simulink model "sim"  (R2020a)
settings: Solver=FixedStepAuto  StartTime=0.0  StopTime=2  FixedStep=0.001  RelTol=1e-3
undefined symbols (not defined in the file): A, B, C, x_0
libraries: simulink_extras x3
settings Model: Creator=Artis  LastModifiedBy=Emil

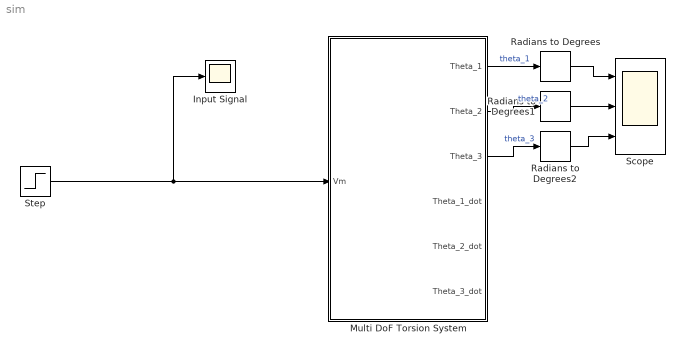
== system sim ==
  Input Signal : Scope
  Multi DoF Torsion System : Subsystem
  Radians to Degrees : simulink_extras/Transformations/Radians to Degrees
  Radians to Degrees1 : simulink_extras/Transformations/Radians to Degrees
  Radians to Degrees2 : simulink_extras/Transformations/Radians to Degrees
  Scope : Scope  NumInputPorts=3
  Step : Step  Before=6  After=0  SampleTime=0
  wires:
  Step/1 -> Multi DoF Torsion System/1(Vm), Input Signal/1
  Radians to Degrees2/1 -> Scope/3
  Radians to Degrees1/1 -> Scope/2
  Radians to Degrees/1 -> Scope/1
  Multi DoF Torsion System/1(Theta_1) -> Radians to Degrees/1  "theta_1"
  Multi DoF Torsion System/2(Theta_2) -> Radians to Degrees1/1  "theta_2"
  Multi DoF Torsion System/3(Theta_3) -> Radians to Degrees2/1  "theta_3"

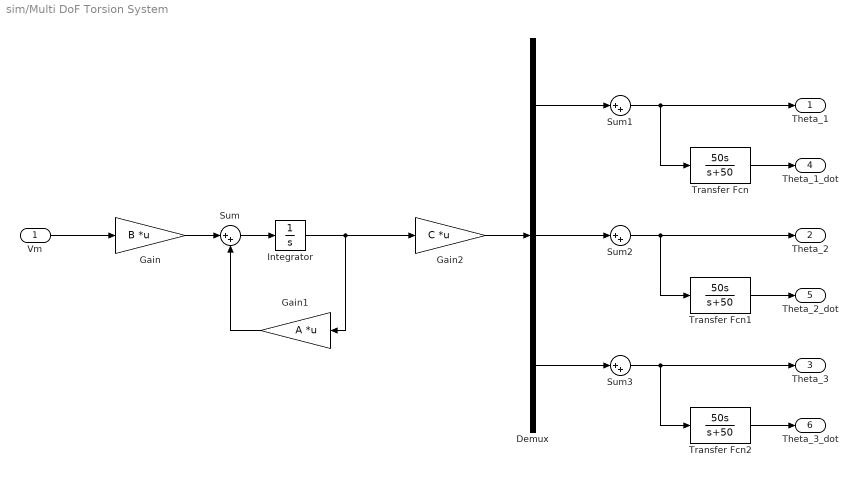
== system sim/Multi DoF Torsion System ==
  Vm : Inport
  Demux : Demux  Outputs=3
  Gain : Gain  Gain=B  Multiplication=Matrix(K*u) (u vector)
  Gain1 : Gain  Gain=A  Multiplication=Matrix(K*u) (u vector)
  Gain2 : Gain  Gain=C  Multiplication=Matrix(K*u) (u vector)
  Integrator : Integrator  InitialCondition=x_0
  Sum{,1..3} (4 alike) : Sum  Inputs=|++
  Transfer Fcn : TransferFcn  Numerator=[50 0]  Denominator=[1 50]
  Transfer Fcn1 : TransferFcn  Numerator=[50 0]  Denominator=[1 50]
  Transfer Fcn2 : TransferFcn  Numerator=[50 0]  Denominator=[1 50]
  Theta_1 : Outport
  Theta_2 : Outport  Port=2
  Theta_3 : Outport  Port=3
  Theta_1_dot : Outport  Port=4
  Theta_2_dot : Outport  Port=5
  Theta_3_dot : Outport  Port=6
  wires:
  Gain/1 -> Sum/1
  Sum/1 -> Integrator/1
  Integrator/1 -> Gain2/1, Gain1/1
  Gain1/1 -> Sum/2
  Gain2/1 -> Demux/1
  Demux/1 -> Sum1/1
  Vm/1 -> Gain/1
  Sum1/1 -> Transfer Fcn/1, Theta_1/1
  Transfer Fcn/1 -> Theta_1_dot/1
  ? -> Sum1/2
  Transfer Fcn1/1 -> Theta_2_dot/1
  ? -> Sum2/2
  Sum2/1 -> Theta_2/1, Transfer Fcn1/1
  Demux/2 -> Sum2/1
  Sum3/1 -> Theta_3/1, Transfer Fcn2/1
  ? -> Sum3/2
  Transfer Fcn2/1 -> Theta_3_dot/1
  Demux/3 -> Sum3/1
